simulink model "model_regulator5"  (R2024a)
settings: Solver=FixedStepAuto  StartTime=0.0  StopTime=10.0  FixedStep=0.01  RelTol=1e-3
undefined symbols (not defined in the file): k_i, k_p
settings Model: Creator=main  LastModifiedBy=main

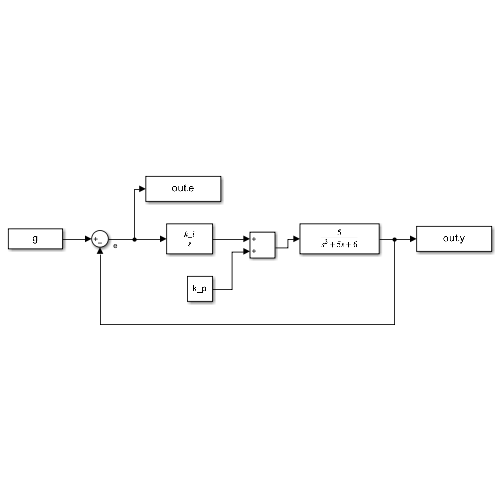
[thumbnail: Simulink's stored preview of the top-level diagram]
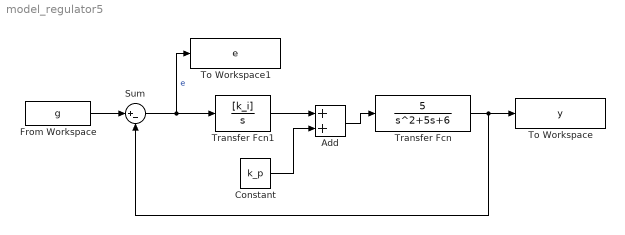
== system model_regulator5 ==
  Add : Sum
  Constant : Constant  Value=k_p
  From Workspace : FromWorkspace  VariableName=g
  Sum : Sum  Inputs=|+-
  To Workspace : ToWorkspace  VariableName=y  SaveFormat=Timeseries  SampleTime=-1
  To Workspace1 : ToWorkspace  VariableName=e  SaveFormat=Timeseries  SampleTime=-1
  Transfer Fcn : TransferFcn  Numerator=[5]  Denominator=[1 5 6]
  Transfer Fcn1 : TransferFcn  Numerator=[k_i]  Denominator=[1 0]
  wires:
  Transfer Fcn/1 -> To Workspace/1, Sum/2
  From Workspace/1 -> Sum/1
  Sum/1 -> Transfer Fcn1/1, To Workspace1/1  "e"
  Transfer Fcn1/1 -> Add/1
  Add/1 -> Transfer Fcn/1
  Constant/1 -> Add/2
